simulink model "mirko_LQR_NL"  (R2025b)
settings: Solver=ode4  StartTime=0.0  StopTime=120  FixedStep=1/10  RelTol=1e-3
undefined symbols (not defined in the file or in its folder): att_alt, Gintlat, GintLong, GintLong_Alt, GstateLat, GstateLong, GstateLong_Alt, Ue, Ve
libraries: simulink_extras x8
settings Model: Creator=anade  LastModifiedBy=kauemartinsdesouza

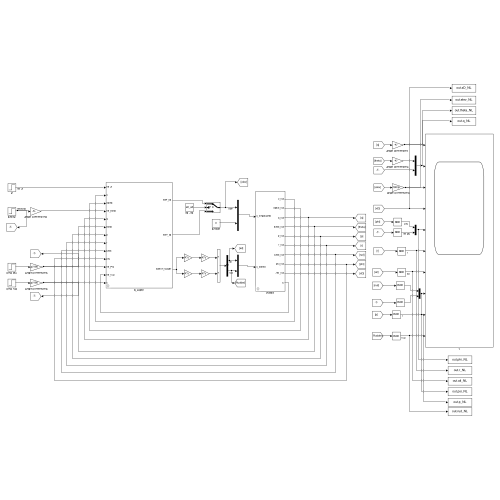
[thumbnail: Simulink's stored preview of the top-level diagram]
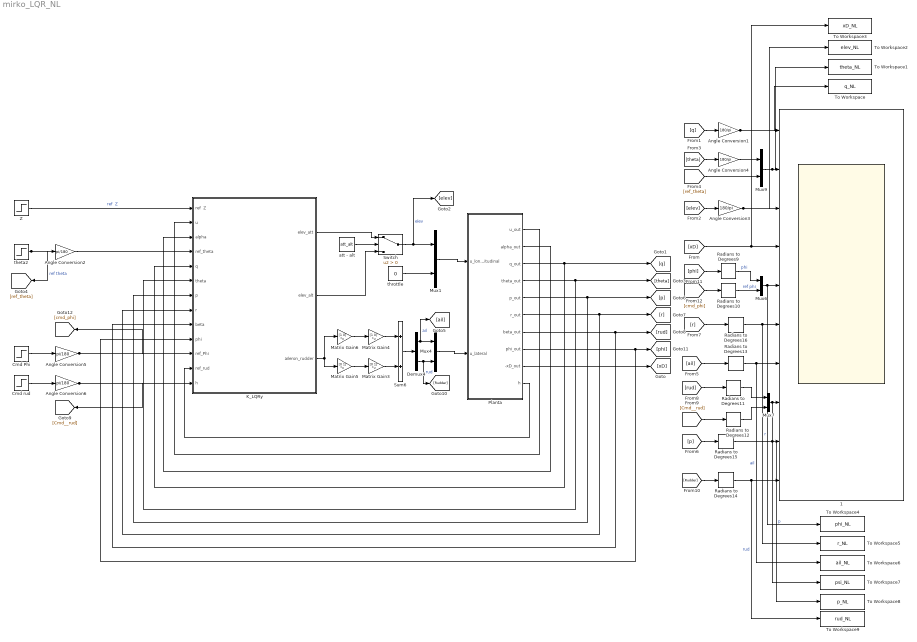
== system mirko_LQR_NL ==
  " 1" : Scope  NumInputPorts=10
      settings: ActiveDisplayString=10  DataLoggingVariableName=ScopeData4
  " Z " : Step  Time=5  After=0  SampleTime=0
  Angle Conversion1 : Gain  Gain=180/pi
  Angle Conversion2 : Gain  Gain=pi/180
  Angle Conversion3 : Gain  Gain=180/pi
  Angle Conversion4 : Gain  Gain=180/pi
  Angle Conversion5 : Gain  Gain=pi/180
  Angle Conversion6 : Gain  Gain=pi/180
  Cmd Phi : Step  Time=30  After=5  SampleTime=0
  Cmd rud : Step  Time=10  After=0  SampleTime=0
  Demux4 : Demux  Outputs=2
      settings: DisplayOption=none
  K_LQRy : Subsystem
  Matrix Gain3 : Gain  Gain=[0 1]'  Multiplication=Matrix(K*u)  SaturateOnIntegerOverflow=on  OutDataTypeStr=Inherit: Same as input  ParamDataTypeStr=Inherit: Same as input
  Matrix Gain4 : Gain  Gain=[1 0]'  Multiplication=Matrix(K*u)  SaturateOnIntegerOverflow=on  OutDataTypeStr=Inherit: Same as input  ParamDataTypeStr=Inherit: Same as input
  Matrix Gain5 : Gain  Gain=[0 1]  Multiplication=Matrix(K*u)  SaturateOnIntegerOverflow=on  OutDataTypeStr=Inherit: Same as input  ParamDataTypeStr=Inherit: Same as input
  Matrix Gain6 : Gain  Gain=[1 0]  Multiplication=Matrix(K*u)  SaturateOnIntegerOverflow=on  OutDataTypeStr=Inherit: Same as input  ParamDataTypeStr=Inherit: Same as input
  Mux{1,4,6..7,9} (5 alike) : Mux  Inputs=2
  Planta : Subsystem
  Radians to Degrees{9..16} (8 alike) : simulink_extras/Transformations/Radians to Degrees
  Sum6 : Sum  Inputs=2  SaturateOnIntegerOverflow=on
  Switch : Switch  Criteria=u2 > Threshold  SaturateOnIntegerOverflow=off  InputSameDT=off
  To Workspace : ToWorkspace  VariableName=q_NL  SaveFormat=Structure With Time  SampleTime=-1
  To Workspace1 : ToWorkspace  VariableName=theta_NL  SaveFormat=Structure With Time  SampleTime=-1
  To Workspace2 : ToWorkspace  VariableName=elev_NL  SaveFormat=Structure With Time  SampleTime=-1
  To Workspace3 : ToWorkspace  VariableName=xD_NL  SaveFormat=Structure With Time  SampleTime=-1
  To Workspace4 : ToWorkspace  VariableName=phi_NL  SaveFormat=Structure With Time  SampleTime=-1
  To Workspace5 : ToWorkspace  VariableName=r_NL  SaveFormat=Structure With Time  SampleTime=-1
  To Workspace6 : ToWorkspace  VariableName=ail_NL  SaveFormat=Structure With Time  SampleTime=-1
  To Workspace7 : ToWorkspace  VariableName=psi_NL  SaveFormat=Structure With Time  SampleTime=-1
  To Workspace8 : ToWorkspace  VariableName=p_NL  SaveFormat=Structure With Time  SampleTime=-1
  To Workspace9 : ToWorkspace  VariableName=rud_NL  SaveFormat=Structure With Time  SampleTime=-1
  att - alt : Constant  Value=att_alt
  theta2 : Step  Time=5  After=5  SampleTime=0
  throttle : Constant  Value=0
  wires:
  Mux9/1 -> To Workspace1/1, " 1"/2
  theta2/1 -> [ref_theta], Angle Conversion2/1  "ref theta"
  Radians to Degrees13/1 -> To Workspace6/1, " 1"/7  "ail"
  Demux4/2 -> Mux4/2, [Rudder]  "rud"
  Radians to Degrees11/1 -> Mux7/1
  Radians to Degrees15/1 -> To Workspace8/1, " 1"/9  "p"
  Matrix Gain5/1 -> Matrix Gain3/1
  Matrix Gain4/1 -> Sum6/1
  Radians to Degrees9/1 -> Mux6/1  "phi"
  Matrix Gain3/1 -> Sum6/2
  Mux6/1 -> " 1"/5, To Workspace4/1
  Matrix Gain6/1 -> Matrix Gain4/1
  Sum6/1 -> Demux4/1
  Radians to Degrees10/1 -> Mux6/2  "ref phi"
  Radians to Degrees14/1 -> To Workspace9/1, " 1"/10  "rud"
  Mux7/1 -> To Workspace7/1, " 1"/8
  Radians to Degrees12/1 -> Mux7/2
  Radians to Degrees16/1 -> To Workspace5/1, " 1"/6  "r"
  Demux4/1 -> [ail], Mux4/1  "ail"
  [xD] -> " 1"/4, To Workspace3/1
  [ref_theta] -> Mux9/2
  [ail] -> Radians to Degrees13/1
  [p] -> Radians to Degrees15/1
  [r] -> Radians to Degrees16/1
  [rud] -> Radians to Degrees11/1
  [Cmd__rud] -> Radians to Degrees12/1
  [Rudder] -> Radians to Degrees14/1
  [phi] -> Radians to Degrees9/1
  [cmd_phi] -> Radians to Degrees10/1
  Switch/1 -> [elev], Mux1/1  "elev"
  throttle/1 -> Mux1/2
  Planta/7(beta_out) -> K_LQRy/9(beta), [rud]
  Planta/5(p_out) -> K_LQRy/7(p), [p]
  Planta/3(q_out) -> K_LQRy/5(q), [q]
  Planta/4(theta_out) -> K_LQRy/6(theta), [theta]
  Planta/8(phi_out) -> K_LQRy/10(phi), [phi]
  Planta/6(r_out) -> K_LQRy/8(r), [r]
  Mux1/1 -> Planta/1(u_longitudinal)
  Mux4/1 -> Planta/2(u_lateral)
  Planta/9(-xD_out) -> [xD]
  K_LQRy/3(aileron_rudder) -> Matrix Gain6/1, Matrix Gain5/1
  " Z "/1 -> K_LQRy/1(ref  Z)  "ref  Z"
  Planta/1(u_out) -> K_LQRy/2(u)
  Planta/2(alpha_out) -> K_LQRy/3(alpha)
  Planta/10(h) -> K_LQRy/13("h ")
  K_LQRy/1(elev_att) -> Switch/1
  K_LQRy/2(elev_alt) -> Switch/3
  att - alt/1 -> Switch/2
  [q] -> Angle Conversion1/1
  Angle Conversion1/1 -> To Workspace/1, " 1"/1
  Angle Conversion2/1 -> K_LQRy/4(ref_theta)
  [elev] -> Angle Conversion3/1
  Angle Conversion3/1 -> " 1"/3, To Workspace2/1
  [theta] -> Angle Conversion4/1
  Angle Conversion4/1 -> Mux9/1
  Cmd Phi/1 -> Angle Conversion5/1
  Angle Conversion5/1 -> K_LQRy/11(ref_Phi), [cmd_phi]
  Cmd rud/1 -> Angle Conversion6/1
  Angle Conversion6/1 -> K_LQRy/12(ref_rud), [Cmd__rud]

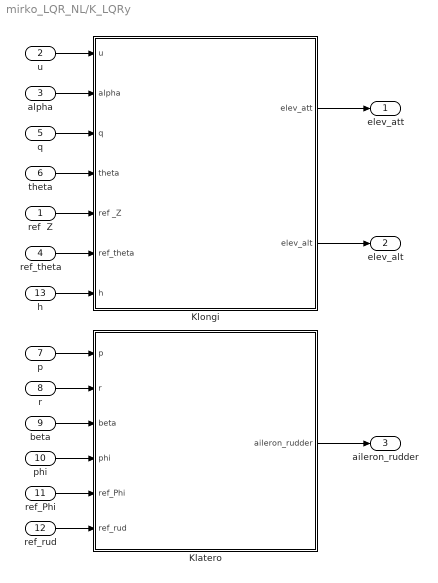
== system mirko_LQR_NL/K_LQRy ==
  ref  Z : Inport
  u : Inport  Port=2
  alpha : Inport  Port=3
  ref_theta : Inport  Port=4
  q : Inport  Port=5
  theta : Inport  Port=6
  p : Inport  Port=7
  r : Inport  Port=8
  beta : Inport  Port=9
  phi : Inport  Port=10
  ref_Phi : Inport  Port=11
  ref_rud : Inport  Port=12
  "h " : Inport  Port=13
  Klatero : Subsystem
  Klongi : Subsystem
  elev_att : Outport
  elev_alt : Outport  Port=2
  aileron_rudder : Outport  Port=3
  wires:
  p/1 -> Klatero/1(p)
  theta/1 -> Klongi/4(theta)
  phi/1 -> Klatero/4(phi)
  u/1 -> Klongi/1(u)
  r/1 -> Klatero/2(r)
  q/1 -> Klongi/3(q)
  beta/1 -> Klatero/3(beta)
  "h "/1 -> Klongi/7("h ")
  ref  Z/1 -> Klongi/5(ref _Z)
  Klatero/1(aileron_rudder) -> aileron_rudder/1
  ref_theta/1 -> Klongi/6(ref_theta)
  alpha/1 -> Klongi/2(alpha)
  ref_rud/1 -> Klatero/6(ref_rud)
  Klongi/1(elev_att) -> elev_att/1
  Klongi/2(elev_alt) -> elev_alt/1
  ref_Phi/1 -> Klatero/5(ref_Phi)

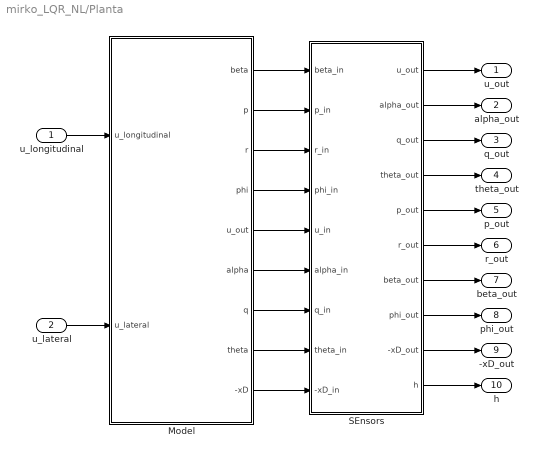
== system mirko_LQR_NL/Planta ==
  u_longitudinal : Inport
  u_lateral : Inport  Port=2
  Model : Subsystem
  SEnsors : Subsystem
  u_out : Outport
  alpha_out : Outport  Port=2
  q_out : Outport  Port=3
  theta_out : Outport  Port=4
  p_out : Outport  Port=5
  r_out : Outport  Port=6
  beta_out : Outport  Port=7
  phi_out : Outport  Port=8
  -xD_out : Outport  Port=9
  h : Outport  Port=10
  wires:
  SEnsors/2(alpha_out) -> alpha_out/1
  SEnsors/3(q_out) -> q_out/1
  SEnsors/1(u_out) -> u_out/1
  Model/7(q) -> SEnsors/7(q_in)
  SEnsors/5(p_out) -> p_out/1
  Model/8(theta) -> SEnsors/8(theta_in)
  SEnsors/4(theta_out) -> theta_out/1
  u_lateral/1 -> Model/2(u_lateral)
  Model/1(beta) -> SEnsors/1(beta_in)
  SEnsors/6(r_out) -> r_out/1
  SEnsors/7(beta_out) -> beta_out/1
  Model/4(phi) -> SEnsors/4(phi_in)
  Model/5(u_out) -> SEnsors/5(u_in)
  SEnsors/9(-xD_out) -> -xD_out/1
  Model/2(p) -> SEnsors/2(p_in)
  Model/9("-xD ") -> SEnsors/9(-xD_in)
  SEnsors/8(phi_out) -> phi_out/1
  Model/3(r) -> SEnsors/3(r_in)
  u_longitudinal/1 -> Model/1(u_longitudinal)
  Model/6(alpha) -> SEnsors/6(alpha_in)
  SEnsors/10(h) -> h/1

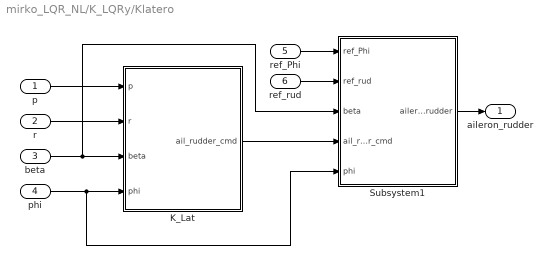
== system mirko_LQR_NL/K_LQRy/Klatero ==
  p : Inport
  r : Inport  Port=2
  beta : Inport  Port=3
  phi : Inport  Port=4
  ref_Phi : Inport  Port=5
  ref_rud : Inport  Port=6
  K_Lat : Subsystem
  Subsystem1 : Subsystem
  aileron_rudder : Outport
  wires:
  K_Lat/1(ail_rudder_cmd) -> Subsystem1/4(ail_rudder_cmd)
  ref_rud/1 -> Subsystem1/2(ref_rud)
  r/1 -> K_Lat/2(r)
  ref_Phi/1 -> Subsystem1/1(ref_Phi)
  beta/1 -> K_Lat/3(beta), Subsystem1/3(beta)
  p/1 -> K_Lat/1(p)
  phi/1 -> K_Lat/4(phi), Subsystem1/5(phi)
  Subsystem1/1(aileron_rudder) -> aileron_rudder/1

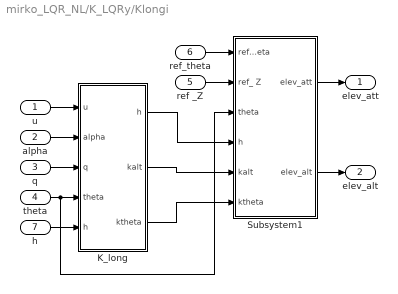
== system mirko_LQR_NL/K_LQRy/Klongi ==
  u : Inport
  alpha : Inport  Port=2
  q : Inport  Port=3
  theta : Inport  Port=4
  ref _Z : Inport  Port=5
  ref_theta : Inport  Port=6
  "h " : Inport  Port=7
  K_long : Subsystem
  Subsystem1 : Subsystem
  elev_att : Outport
  elev_alt : Outport  Port=2
  wires:
  ref_theta/1 -> Subsystem1/1(ref_theta)
  u/1 -> K_long/1(u)
  K_long/2(kalt) -> Subsystem1/5(kalt)
  K_long/1(h) -> Subsystem1/4(h)
  alpha/1 -> K_long/2(alpha)
  q/1 -> K_long/3(q)
  ref _Z/1 -> Subsystem1/2(ref_ Z)
  Subsystem1/1(elev_att) -> elev_att/1
  K_long/3(ktheta) -> Subsystem1/6(ktheta)
  Subsystem1/2(elev_alt) -> elev_alt/1
  theta/1 -> K_long/4(theta), Subsystem1/3(theta)
  "h "/1 -> K_long/5("h ")

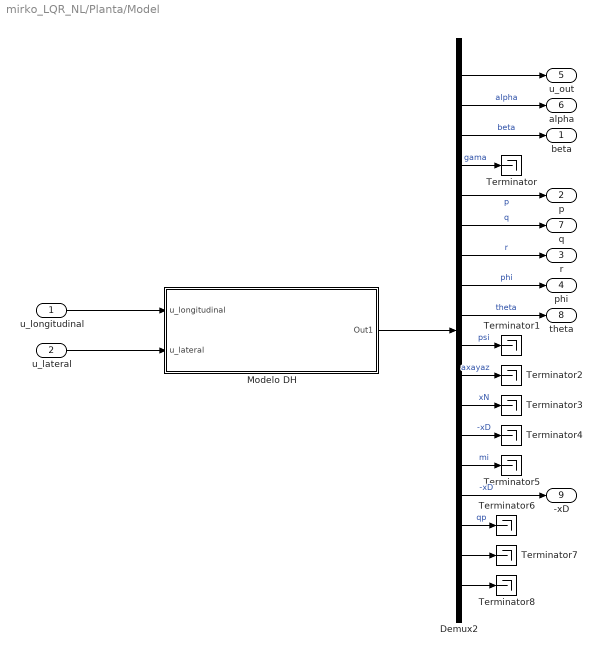
== system mirko_LQR_NL/Planta/Model ==
  u_longitudinal : Inport
  u_lateral : Inport  Port=2
  Demux2 : Demux  Outputs=18
  Modelo DH : Subsystem
  Terminator{,1..8} (9 alike) : Terminator
  beta : Outport
  p : Outport  Port=2
  r : Outport  Port=3
  phi : Outport  Port=4
  u_out : Outport  Port=5
  alpha : Outport  Port=6
  q : Outport  Port=7
  theta : Outport  Port=8
  "-xD " : Outport  Port=9
  wires:
  Demux2/9 -> theta/1  "theta"
  u_longitudinal/1 -> Modelo DH/1(u_longitudinal)
  Demux2/3 -> beta/1  "beta"
  Demux2/5 -> p/1  "p"
  Demux2/7 -> r/1  "r"
  Demux2/1 -> u_out/1
  Demux2/2 -> alpha/1  "alpha"
  Demux2/8 -> phi/1  "phi"
  Modelo DH/1(Out1) -> Demux2/1
  Demux2/15 -> "-xD "/1  "-xD"
  Demux2/6 -> q/1  "q"
  u_lateral/1 -> Modelo DH/2(u_lateral)
  Demux2/4 -> Terminator/1  "gama"
  Demux2/10 -> Terminator1/1  "psi"
  Demux2/11 -> Terminator2/1  "axayaz"
  Demux2/12 -> Terminator3/1  "xN"
  Demux2/13 -> Terminator4/1  "-xD"
  Demux2/14 -> Terminator5/1  "mi"
  Demux2/16 -> Terminator6/1  "qp"
  Demux2/17 -> Terminator7/1
  Demux2/18 -> Terminator8/1

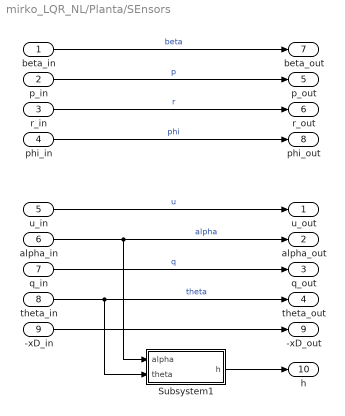
== system mirko_LQR_NL/Planta/SEnsors ==
  beta_in : Inport
  p_in : Inport  Port=2
  r_in : Inport  Port=3
  phi_in : Inport  Port=4
  u_in : Inport  Port=5
  alpha_in : Inport  Port=6
  q_in : Inport  Port=7
  theta_in : Inport  Port=8
  -xD_in : Inport  Port=9
  Subsystem1 : Subsystem
  u_out : Outport
  alpha_out : Outport  Port=2
  q_out : Outport  Port=3
  theta_out : Outport  Port=4
  p_out : Outport  Port=5
  r_out : Outport  Port=6
  beta_out : Outport  Port=7
  phi_out : Outport  Port=8
  -xD_out : Outport  Port=9
  h : Outport  Port=10
  wires:
  p_in/1 -> p_out/1  "p"
  phi_in/1 -> phi_out/1  "phi"
  r_in/1 -> r_out/1  "r"
  alpha_in/1 -> alpha_out/1, Subsystem1/1(alpha)  "alpha"
  beta_in/1 -> beta_out/1  "beta"
  u_in/1 -> u_out/1  "u"
  q_in/1 -> q_out/1  "q"
  theta_in/1 -> theta_out/1, Subsystem1/2(theta)  "theta"
  -xD_in/1 -> -xD_out/1
  Subsystem1/1(h) -> h/1

== system mirko_LQR_NL/K_LQRy/Klatero/K_Lat ==
  p : Inport
  r : Inport  Port=2
  beta : Inport  Port=3
  phi : Inport  Port=4
  Mux5 : Mux
  states1 : Gain  Gain=GstateLat  Multiplication=Matrix(K*u)  SaturateOnIntegerOverflow=on  OutDataTypeStr=Inherit: Same as input  ParamDataTypeStr=Inherit: Same as input
  ail_rudder_cmd : Outport
  wires:
  Mux5/1 -> states1/1
  phi/1 -> Mux5/4
  p/1 -> Mux5/2
  states1/1 -> ail_rudder_cmd/1  "ail cmd, rudder cmd"
  r/1 -> Mux5/3
  beta/1 -> Mux5/1

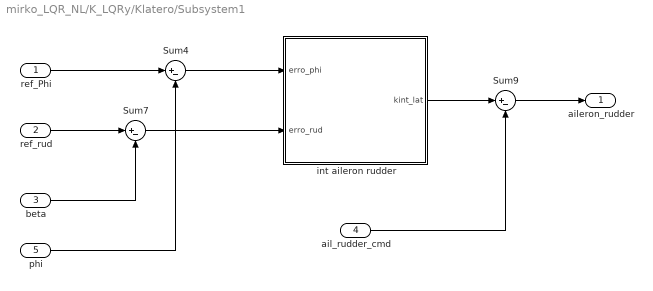
== system mirko_LQR_NL/K_LQRy/Klatero/Subsystem1 ==
  ref_Phi : Inport
  ref_rud : Inport  Port=2
  beta : Inport  Port=3
  ail_rudder_cmd : Inport  Port=4
  phi : Inport  Port=5
  Sum4 : Sum  Inputs=|+-  SaturateOnIntegerOverflow=on
  Sum7 : Sum  Inputs=|+-  SaturateOnIntegerOverflow=on
  Sum9 : Sum  Inputs=|+-  SaturateOnIntegerOverflow=on
  int aileron rudder : Subsystem
  aileron_rudder : Outport
  wires:
  Sum7/1 -> int aileron rudder/2(erro_rud)
  Sum4/1 -> int aileron rudder/1(erro_phi)
  ref_rud/1 -> Sum7/1
  int aileron rudder/1(kint_lat) -> Sum9/1
  phi/1 -> Sum4/2
  ail_rudder_cmd/1 -> Sum9/2
  ref_Phi/1 -> Sum4/1
  Sum9/1 -> aileron_rudder/1
  beta/1 -> Sum7/2

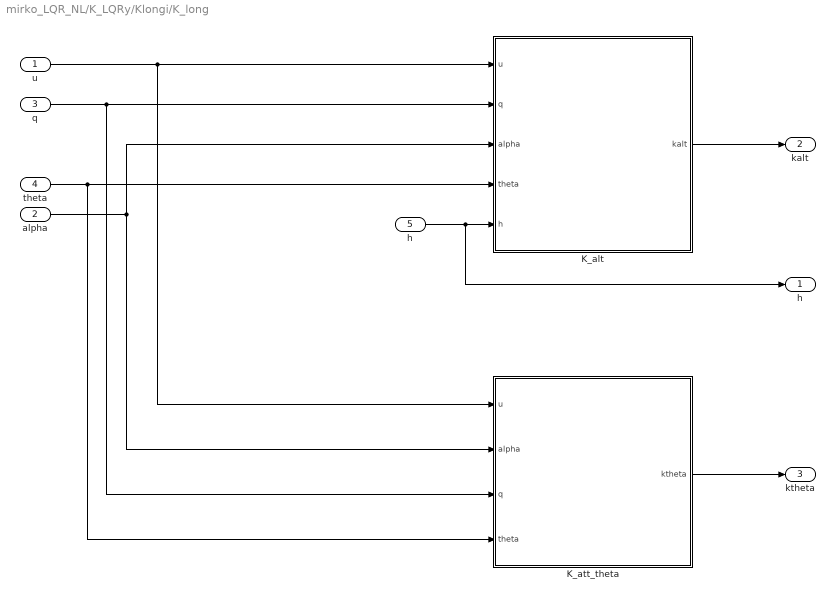
== system mirko_LQR_NL/K_LQRy/Klongi/K_long ==
  u : Inport
  alpha : Inport  Port=2
  q : Inport  Port=3
  theta : Inport  Port=4
  "h " : Inport  Port=5
  K_alt : Subsystem
  K_att_theta : Subsystem
  h : Outport
  kalt : Outport  Port=2
  ktheta : Outport  Port=3
  wires:
  theta/1 -> K_att_theta/4(theta), K_alt/4(theta)
  q/1 -> K_alt/2(q), K_att_theta/3(q)
  K_att_theta/1(ktheta) -> ktheta/1
  u/1 -> K_alt/1(u), K_att_theta/1(u)
  K_alt/1(kalt) -> kalt/1
  "h "/1 -> h/1, K_alt/5(h)
  alpha/1 -> K_att_theta/2(alpha), K_alt/3(alpha)

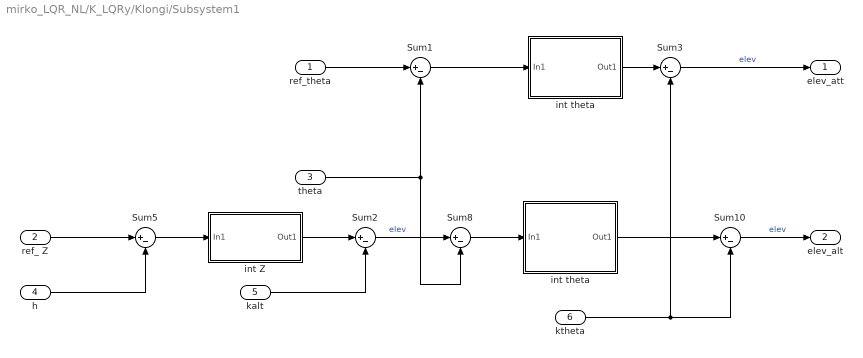
== system mirko_LQR_NL/K_LQRy/Klongi/Subsystem1 ==
  ref_theta : Inport
  ref_ Z : Inport  Port=2
  theta : Inport  Port=3
  h : Inport  Port=4
  kalt : Inport  Port=5
  ktheta : Inport  Port=6
  Sum{1..3,5,8,10} (6 alike) : Sum  Inputs=|+-
  int Z : Subsystem
  int theta : Subsystem
  "int theta " : Subsystem
  elev_att : Outport
  elev_alt : Outport  Port=2
  wires:
  kalt/1 -> Sum2/2
  theta/1 -> Sum8/2, Sum1/2
  int Z/1(Out1) -> Sum2/1
  ref_ Z/1 -> Sum5/1
  Sum1/1 -> int theta/1(In1)
  h/1 -> Sum5/2
  Sum10/1 -> elev_alt/1  "elev"
  int theta/1(Out1) -> Sum3/1
  Sum3/1 -> elev_att/1  "elev"
  ktheta/1 -> Sum3/2, Sum10/2
  ref_theta/1 -> Sum1/1
  Sum8/1 -> "int theta "/1(In1)
  "int theta "/1(Out1) -> Sum10/1
  Sum2/1 -> Sum8/1  "elev"
  Sum5/1 -> int Z/1(In1)

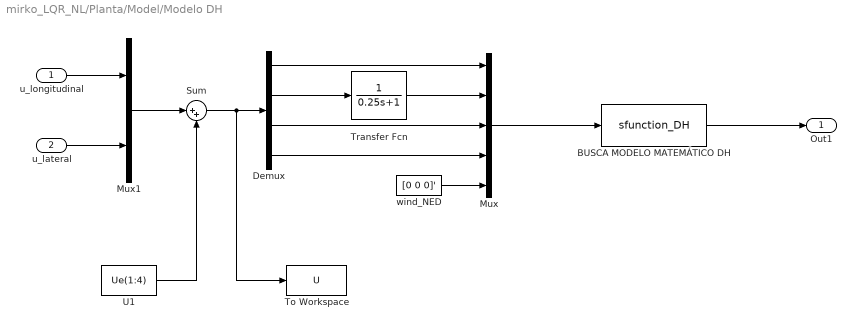
== system mirko_LQR_NL/Planta/Model/Modelo DH ==
  u_longitudinal : Inport
  u_lateral : Inport  Port=2
  "BUSCA MODELO MATEMÁTICO DH " : S-Function  FunctionName=sfunction_DH  Parameters=Xe, coef_Sato, coef_Ana  SFunctionDeploymentMode=off  EnableBusSupport=off
  Demux : Demux
  Mux : Mux  Inputs=5
  Mux1 : Mux  Inputs=2
  Sum : Sum  Inputs=|++
  To Workspace : ToWorkspace  VariableName=U  SampleTime=-1
  Transfer Fcn : TransferFcn  Denominator=[0.25 1]
  U1 : Constant  Value=Ue(1:4)
  wind_NED : Constant  Value=[0 0 0]'
  Out1 : Outport
  wires:
  Transfer Fcn/1 -> Mux/2
  Demux/1 -> Mux/1
  "BUSCA MODELO MATEMÁTICO DH "/1 -> Out1/1
  Demux/4 -> Mux/4
  Demux/3 -> Mux/3
  Demux/2 -> Transfer Fcn/1
  Mux/1 -> "BUSCA MODELO MATEMÁTICO DH "/1
  Mux1/1 -> Sum/1
  Sum/1 -> To Workspace/1, Demux/1
  U1/1 -> Sum/2
  u_lateral/1 -> Mux1/2
  u_longitudinal/1 -> Mux1/1
  wind_NED/1 -> Mux/5

== system mirko_LQR_NL/Planta/SEnsors/Subsystem1 ==
  alpha : Inport
  theta : Inport  Port=2
  Add : Sum  Inputs=-+
  Gain : Gain  Gain=Ve
  Integrator2 : Integrator
  h : Outport
  wires:
  Add/1 -> Gain/1
  Integrator2/1 -> h/1
  Gain/1 -> Integrator2/1
  alpha/1 -> Add/1
  theta/1 -> Add/2

== system mirko_LQR_NL/K_LQRy/Klatero/Subsystem1/int aileron rudder ==
  erro_phi : Inport
  erro_rud : Inport  Port=2
  Integrator1 : Integrator
  Integrator4 : Integrator
  Mux10 : Mux  Inputs=2
  int : Gain  Gain=Gintlat  Multiplication=Matrix(K*u)  SaturateOnIntegerOverflow=on  OutDataTypeStr=Inherit: Same as input  ParamDataTypeStr=Inherit: Same as input
  kint_lat : Outport
  wires:
  Integrator1/1 -> Mux10/2
  Integrator4/1 -> Mux10/1
  int/1 -> kint_lat/1
  Mux10/1 -> int/1
  erro_phi/1 -> Integrator4/1
  erro_rud/1 -> Integrator1/1

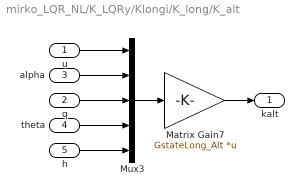
== system mirko_LQR_NL/K_LQRy/Klongi/K_long/K_alt ==
  u : Inport
  q : Inport  Port=2
  alpha : Inport  Port=3
  theta : Inport  Port=4
  h : Inport  Port=5
  Matrix Gain7 : Gain  Gain=GstateLong_Alt  Multiplication=Matrix(K*u)  SaturateOnIntegerOverflow=on  OutDataTypeStr=Inherit: Same as input  ParamDataTypeStr=Inherit: Same as input
  Mux3 : Mux  Inputs=5
  kalt : Outport
  wires:
  Mux3/1 -> Matrix Gain7/1
  h/1 -> Mux3/5
  u/1 -> Mux3/1
  q/1 -> Mux3/3
  alpha/1 -> Mux3/2
  theta/1 -> Mux3/4
  Matrix Gain7/1 -> kalt/1

== system mirko_LQR_NL/K_LQRy/Klongi/K_long/K_att_theta ==
  u : Inport
  alpha : Inport  Port=2
  q : Inport  Port=3
  theta : Inport  Port=4
  Matrix Gain1 : Gain  Gain=GstateLong  Multiplication=Matrix(K*u)  SaturateOnIntegerOverflow=on  OutDataTypeStr=Inherit: Same as input  ParamDataTypeStr=Inherit: Same as input
  Mux2 : Mux
  ktheta : Outport
  wires:
  Mux2/1 -> Matrix Gain1/1
  q/1 -> Mux2/3
  theta/1 -> Mux2/4
  alpha/1 -> Mux2/2
  u/1 -> Mux2/1
  Matrix Gain1/1 -> ktheta/1

== system mirko_LQR_NL/K_LQRy/Klongi/Subsystem1/int Z ==
  In1 : Inport
  Integrator3 : Integrator
  Matrix Gain8 : Gain  Gain=GintLong_Alt  Multiplication=Matrix(K*u)  SaturateOnIntegerOverflow=on  OutDataTypeStr=Inherit: Same as input  ParamDataTypeStr=Inherit: Same as input
  Out1 : Outport
  wires:
  Integrator3/1 -> Matrix Gain8/1
  In1/1 -> Integrator3/1
  Matrix Gain8/1 -> Out1/1

== system mirko_LQR_NL/K_LQRy/Klongi/Subsystem1/int theta ==
  In1 : Inport
  Integrator : Integrator
  Matrix Gain2 : Gain  Gain=GintLong  Multiplication=Matrix(K*u)  SaturateOnIntegerOverflow=on  OutDataTypeStr=Inherit: Same as input  ParamDataTypeStr=Inherit: Same as input
  Out1 : Outport
  wires:
  Integrator/1 -> Matrix Gain2/1
  In1/1 -> Integrator/1
  Matrix Gain2/1 -> Out1/1

== system mirko_LQR_NL/K_LQRy/Klongi/Subsystem1/int theta  ==
  In1 : Inport
  Integrator5 : Integrator
  Matrix Gain9 : Gain  Gain=GintLong  Multiplication=Matrix(K*u)  SaturateOnIntegerOverflow=on  OutDataTypeStr=Inherit: Same as input  ParamDataTypeStr=Inherit: Same as input
  Out1 : Outport
  wires:
  Integrator5/1 -> Matrix Gain9/1
  Matrix Gain9/1 -> Out1/1
  In1/1 -> Integrator5/1
